simulink model "OpenClosedwithRampIn"  (R2019a)
settings: Solver=VariableStepAuto  StartTime=0.0  StopTime=10.0  RelTol=1e-3
libraries: simulink x6
settings Model: Creator=G5  LastModifiedBy=G5

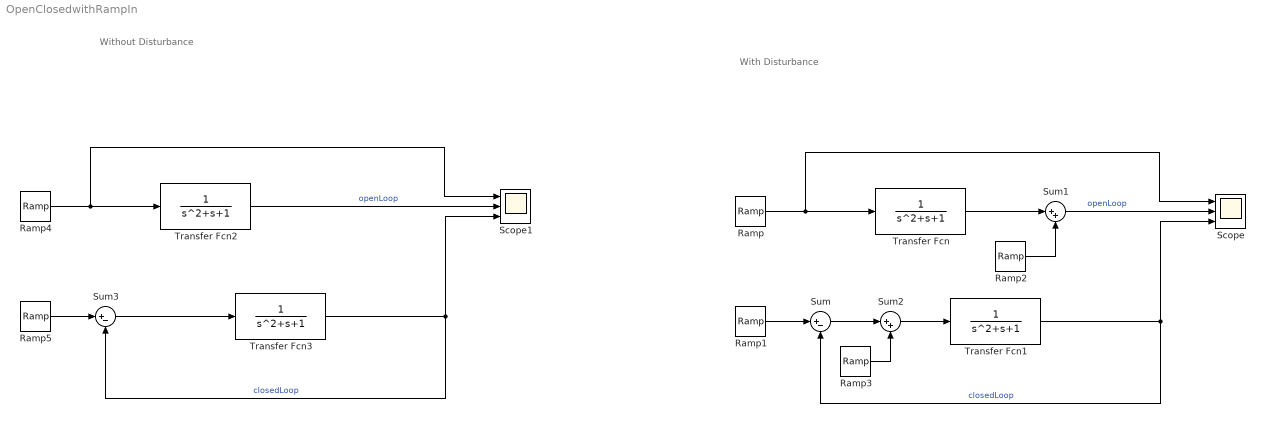
== system OpenClosedwithRampIn ==
  note: With Disturbance
  note: Without Disturbance
  Ramp{,1,4..5} (4 alike) : simulink/Sources/Ramp  slope=1  start=0  InitialOutput=0
  Ramp2 : simulink/Sources/Ramp  slope=0.5  start=0  InitialOutput=0
  Ramp3 : simulink/Sources/Ramp  slope=0.5  start=0  InitialOutput=0
  Scope : Scope  NumInputPorts=3
  Scope1 : Scope  NumInputPorts=3
  Sum : Sum  Inputs=|+-
  Sum1 : Sum  Inputs=|++
  Sum2 : Sum  Inputs=|++
  Sum3 : Sum  Inputs=|+-
  Transfer Fcn{,1..3} (4 alike) : TransferFcn  Denominator=[1 1 1]
  wires:
  Ramp/1 -> Scope/1, Transfer Fcn/1
  Ramp1/1 -> Sum/1
  Transfer Fcn1/1 -> Scope/3, Sum/2  "closedLoop"
  Transfer Fcn/1 -> Sum1/1
  Ramp2/1 -> Sum1/2
  Sum1/1 -> Scope/2  "openLoop"
  Sum/1 -> Sum2/1
  Sum2/1 -> Transfer Fcn1/1
  Ramp3/1 -> Sum2/2
  Sum3/1 -> Transfer Fcn3/1
  Transfer Fcn2/1 -> Scope1/2  "openLoop"
  Transfer Fcn3/1 -> Sum3/2, Scope1/3  "closedLoop"
  Ramp5/1 -> Sum3/1
  Ramp4/1 -> Transfer Fcn2/1, Scope1/1
